simulink model "ARCH_AT51_example"  (R2017b)
settings: Solver=FixedStepAuto  StartTime=0.0  StopTime=10.0  FixedStep=fixedStepSize  RelTol=1e-3
undefined symbols (not defined in the file): fixedStepSize
libraries: simulink x2
settings Model: Creator=JEDDELAN  LastModifiedBy=JEDDELAN
settings DataIOCC: SaveOutput=off  SaveTime=off
settings GRTTargetCC: CombineOutputUpdateFcns=off  MatFileLogging=off

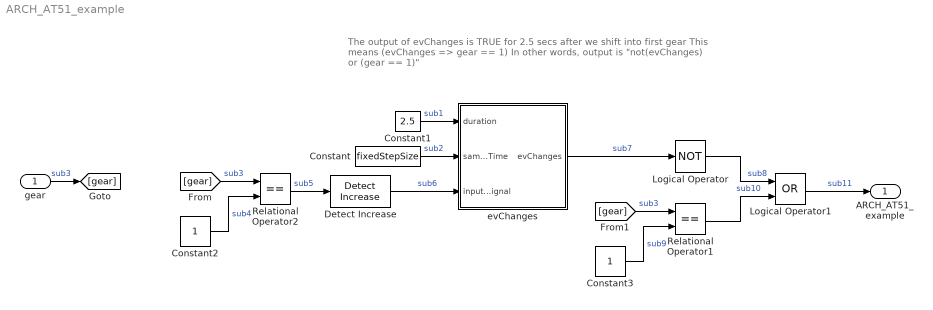
== system ARCH_AT51_example ==
  note: The output of evChanges is TRUE for 2.5 secs after we shift into first gear
      | This means (evChanges => gear == 1)
      | In other words, output is "not(evChanges) or (gear == 1)"
  gear : Inport
  Constant : Constant  Value=fixedStepSize
  Constant1 : Constant  Value=2.5
  Constant2 : Constant
  Constant3 : Constant
  Detect Increase : simulink/Logic and Bit Operations/Detect Increase  vinit=1  OutDataTypeStr=boolean
  Logical Operator : Logic  Operator=NOT  AllPortsSameDT=off  OutDataTypeStr=boolean
  Logical Operator1 : Logic  Operator=OR  AllPortsSameDT=off  OutDataTypeStr=boolean
  Relational Operator1 : RelationalOperator  Operator===  OutDataTypeStr=boolean  RndMeth=Simplest
  Relational Operator2 : RelationalOperator  Operator===  OutDataTypeStr=boolean  RndMeth=Simplest
  evChanges : Subsystem
      settings: CopyFcn=set_param(gcbh,'LinkStatus','none');
  ARCH_AT51_example : Outport  OutDataTypeStr=boolean  PortDimensions=1
  wires:
  gear/1 -> [gear]  "sub3"
  Constant2/1 -> Relational Operator2/2  "sub4"
  Relational Operator2/1 -> Detect Increase/1  "sub5"
  Detect Increase/1 -> evChanges/3(inputSignal)  "sub6"
  evChanges/1(evChanges) -> Logical Operator/1  "sub7"
  Constant/1 -> evChanges/2(sampleTime)  "sub2"
  Constant1/1 -> evChanges/1(duration)  "sub1"
  [gear] -> Relational Operator2/1  "sub3"
  [gear] -> Relational Operator1/1  "sub3"
  Constant3/1 -> Relational Operator1/2  "sub9"
  Relational Operator1/1 -> Logical Operator1/2  "sub10"
  Logical Operator/1 -> Logical Operator1/1  "sub8"
  Logical Operator1/1 -> ARCH_AT51_example/1  "sub11"

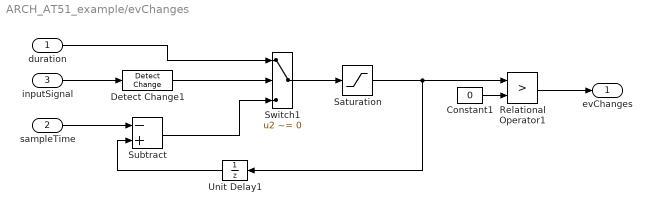
== system ARCH_AT51_example/evChanges ==
  duration : Inport
  sampleTime : Inport  Port=2
  inputSignal : Inport  Port=3
  Constant1 : Constant  Value=0
  Detect Change1 : simulink/Logic and Bit Operations/Detect Change  vinit=0  OutDataTypeStr=boolean
  Relational Operator1 : RelationalOperator  Operator=>  OutDataTypeStr=boolean  RndMeth=Nearest
  Saturation : Saturate  UpperLimit=Inf  LowerLimit=0
  Subtract : Sum  Inputs=-+
  Switch1 : Switch  Criteria=u2 ~= 0
  Unit Delay1 : UnitDelay  SampleTime=-1
  evChanges : Outport
  wires:
  Detect Change1/1 -> Switch1/2
  duration/1 -> Switch1/1
  Switch1/1 -> Saturation/1
  inputSignal/1 -> Detect Change1/1
  Constant1/1 -> Relational Operator1/2
  Subtract/1 -> Switch1/3
  Saturation/1 -> Relational Operator1/1, Unit Delay1/1
  Unit Delay1/1 -> Subtract/2
  Relational Operator1/1 -> evChanges/1
  sampleTime/1 -> Subtract/1
